simulink model "MotorPositionctrl"  (R2020a)
settings: Solver=VariableStepAuto  StartTime=0.0  StopTime=10.0  RelTol=1e-3
undefined symbols (not defined in the file or in its folder): b, J, K, L, R
settings Model: Creator=USER  LastModifiedBy=USER

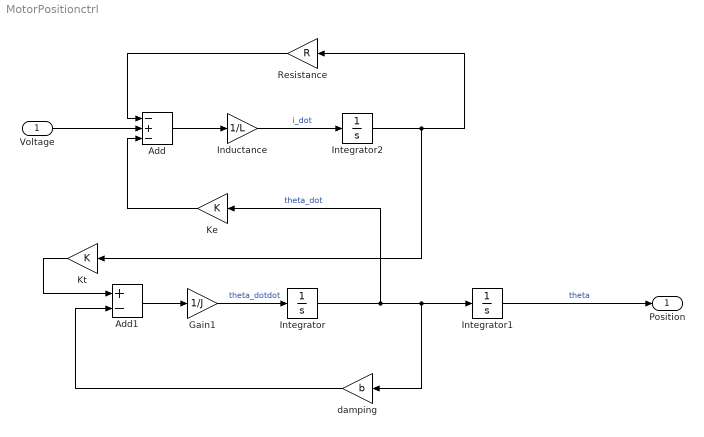
== system MotorPositionctrl ==
  Voltage : Inport
  Add : Sum  Inputs=-+-
  Add1 : Sum  Inputs=+-
  Gain1 : Gain  Gain=1/J
  Inductance : Gain  Gain=1/L
  Integrator : Integrator
  Integrator1 : Integrator
  Integrator2 : Integrator
  Ke : Gain  Gain=K
  Kt : Gain  Gain=K
  Resistance : Gain  Gain=R
  damping : Gain  Gain=b
  Position : Outport
  wires:
  Inductance/1 -> Integrator2/1  "i_dot"
  Gain1/1 -> Integrator/1  "theta_dotdot"
  Add/1 -> Inductance/1
  Resistance/1 -> Add/1
  Add1/1 -> Gain1/1
  damping/1 -> Add1/2
  Integrator/1 -> Ke/1, damping/1, Integrator1/1  "theta_dot"
  Kt/1 -> Add1/1
  Ke/1 -> Add/3
  Voltage/1 -> Add/2
  Integrator1/1 -> Position/1  "theta"
  Integrator2/1 -> Kt/1, Resistance/1
